simulink model "q5"  (R2026a)
settings: Solver=VariableStepAuto
libraries: simulink x1
settings Model: Creator=LAB_PC  LastModifiedBy=LAB_PC

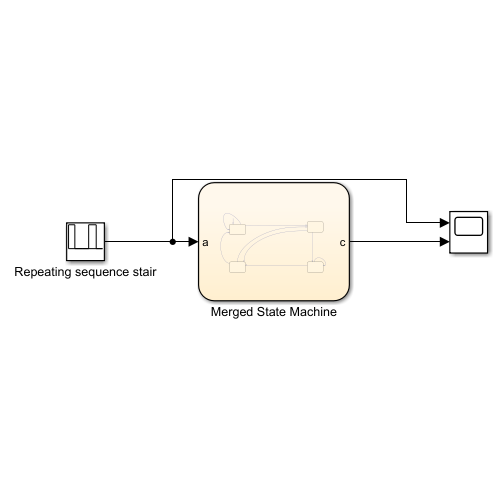
[thumbnail: Simulink's stored preview of the top-level diagram]
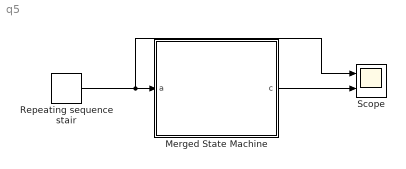
== system q5 ==
  Merged State Machine : Stateflow chart  TreatAsAtomicUnit=on
  Repeating sequence stair : simulink/Sources/Repeating Sequence Stair  OutValues=[1 0 0 1 0]  tsamp=-1  OutMin=[]  OutMax=[]  OutDataTypeStr=double  OutputDataTypeScalingMode=double  OutDataType=fixdt(0,8)  ConRadixGroup=Best Precision: Vector-wise  OutScaling=2^-12
  Scope : Scope  NumInputPorts=2
      settings: ActiveDisplayYMinimum=-0.12499999999999997  ActiveDisplayYMaximum=1.125
  wires:
  Repeating sequence stair/1 -> Scope/1, Merged State Machine/1(a)
  Merged State Machine/1(c) -> Scope/2

== stateflow chart q5/Merged State Machine ==
  state s2_s3
  state s1_s3
  state s2_s4
  state s1_s4
  s1_s3 -> s1_s3 [order 1] : [a == 1] {c = 0;}
  (default) -> s1_s3
  s1_s3 -> s2_s3 [order 2] : [a==0] {c=0;}
  s2_s4 -> s2_s3 [order 1] : [a == 1] {c = 0;}
  s2_s3 -> s2_s4 [order 1] : [a == 1] {c = 1;}
  s2_s4 -> s1_s3 [order 2] : [a == 0] {c = 0;}
  s2_s3 -> s1_s4 [order 2] : [a == 0] {c = 1;}
  s1_s4 -> s1_s4 [order 1] : [a == 1] {c = 1;}
  s1_s4 -> s2_s4 [order 2] : [a == 0] {c = 1;}
  data: a input; c output
